simulink library "CartesianLib"  (R2024a)
settings: Solver=VariableStepAuto  StartTime=0.0  StopTime=10.0  RelTol=1e-3
undefined symbols (not defined in the file): X, Y, Z
libraries: sm_lib x43
(part 1 of 2)
settings Model: Creator=abirdas  LastModifiedBy=abirdas

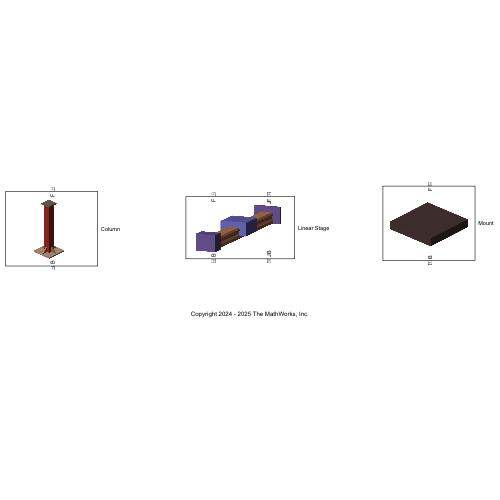
[thumbnail: Simulink's stored preview of the top-level diagram]
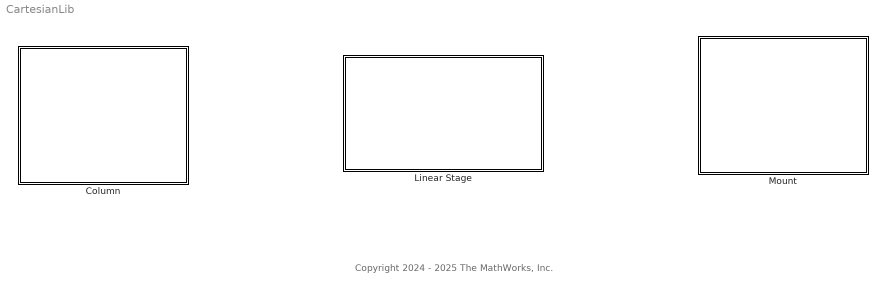
== system CartesianLib ==
  note: Copyright 2024 - 2025 The MathWorks, Inc.
  Column : Subsystem  mask(Column){lengthColumn=0.2, widthColumn=0.02, typeInertiaColumn=Calculate from Geometry, densityColumn=7780, massColumn=1, CMColumn=[0 0 0], MOIColumn=[1 1 1], POIColumn=[0 0 0], colorColumn=[0.8 0.2 0.2]}
      mask prompts: lengthColumn "Column length (m)"; widthColumn "Column width (m)"; typeInertiaColumn "Inertia type"; densityColumn "Density (kg/m^3)"; massColumn "Mass (kg)"; CMColumn "Center of mass (m)"; MOIColumn "Moments of inertia (kg/m^2)"; POIColumn "Products of inertia (kg/m^2)"; colorColumn "Column color"
      mask help:
      | Consists of a bottom plate, a pillar, a top plate and four gusset plates. These components are rigidly connected to one another.
      |
      | Attachment points are:
      | B: Body frame located at the centroid of the bottom surface of the bottom plate of the column.
      | F: Body frame located at the centroid of the top surface of the top plate of the column.
      |
      | Where
      | Column length: Length of the vertical pillar
      | Column width: Width of the vertical pillar
      mask init:
      | % Vertices of gusset plate
      | v1 = [0, 0];
      | v2 = [0.8*widthColumn, 0];
      | v3 = [0, 0.8*widthColumn];
      | sectionGusset = [v1; v2; v3];
      settings: PortSchema="{\"entries\":[{\"content\":{\"sides\":[{\"content\":{},\"type\":\"ConnectorPlacement.EquallySpacedRectSide\",\"uuid\":\"5b485af5-4f05-4248-a7f3-08377bf9cff2\"},{\"content\":{\"side\":\"RIGHT\"},\"type\":\"ConnectorPlacement.EquallySpacedRectSide\",\"uuid\":\"824380b3-967b-4422-aed9-09760effc9b4\"},{\"content\":{\"connectorIds\":[\"LConn1\"],\"side\":\"TOP\"},\"type\":\"ConnectorPlacement.EquallySpacedRectSide\",\"uuid\":\"4c7d634e-a270-49ee-a9b6-ce866eb97663\"},{\"content\":{\"connectorIds\":[\"RConn1\"],\"side\":\"BOTTOM\"},\"type\":\"ConnectorPlacement.EquallySpacedRectSide\",\"uuid\":\"85de5209-dd21-416e-83dd-d7e9fdf0c122\"}]},\"type\":\"ConnectorPlacement.EquallySpacedConnector\",\"uuid\":\"704e5fa1-0bef-4b5b-a1a4-570354550c26\"}],\"packageUris\":[\"http://schema.mathworks.com/mf0/Connector/R2020b\"],\"version\":\"1.0\"}"
      mask Help: web('DocumentationColumn.html')
      mask Callback typeInertiaColumn:
      | maskObj = Simulink.Mask.get(gcb);
      | typeInertiaColumn = maskObj.getParameter('typeInertiaColumn');
      | massColumn = maskObj.getParameter('massColumn');
      | CMColumn = maskObj.getParameter('CMColumn');
      | MOIColumn = maskObj.getParameter('MOIColumn');
      | POIColumn = maskObj.getParameter('POIColumn');
      | densityColumn = maskObj.getParameter('densityColumn');
      | basePlatePath = [gcb,'/Base Plate'];
      | pillarPath = [gcb,'/Pillar'];
      | topPlatePath = [gcb,'/Top Plate'];
      | gusset1Path = [gcb,'/Gusset plate1'];
      | gusset2Path = [gcb,'/Gusset plate2'];
      | gusset3Path = [gcb,'/Gusset plate3'];
      | gusset4Path = [gcb,'/Gusset plate4'];
      | 
      | if strcmp(typeInertiaColumn.Value,'Calculate from Geometry')
      |     massColumn.Visible='off';
      |     CMColumn.Visible='off';
      |     MOIColumn.Visible='off';
      |     POIColumn.Visible='off';
      |     densityColumn.Visible='on';
      |     set_param(basePlatePath,'InertiaType','CalculateFromGeometry');
      |     set_param(basePlatePath,'BasedOnType','Density');
      |     set_param(pillarPath,'InertiaType','CalculateFromGeometry');
      |     set_param(pillarPath,'BasedOnType','Density');
      |     set_param(topPlatePath,'InertiaType','CalculateFromGeometry');
      |     set_param(topPlatePath,'BasedOnType','Density');
      |     set_param(gusset1Path,'InertiaType','CalculateFromGeometry');
      |     set_param(gusset1Path,'BasedOnType','Density');
      |     set_param(gusset2Path,'InertiaType','CalculateFromGeometry');
      |     set_param(gusset2Path,'BasedOnType','Density');
      |     set_param(gusset3Path,'InertiaType','CalculateFromGeometry');
      |     set_param(gusset3Path,'BasedOnType','Density');
      |     set_param(gusset4Path,'InertiaType','CalculateFromGeometry');
      |     set_param(gusset4Path,'BasedOnType','Density');
      | elseif strcmp(typeInertiaColumn.Value,'Custom')
      |     massColumn.Visible='on';
      |     CMColumn.Visible='on';
      |     MOIColumn.Visible='on';
      |     POIColumn.Visible='on';
      |     densityColumn.Visible='off';
      |     set_param(basePlatePath,'InertiaType','Custom');
      |     set_param(pillarPath,'InertiaType','Custom');
      |     set_param(topPlatePath,'InertiaType','Custom');
      |     set_param(gusset1Path,'InertiaType','Custom');
      |     set_param(gusset2Path,'InertiaType','Custom');
      |     set_param(gusset3Path,'InertiaType','Custom');
      |     set_param(gusset4Path,'InertiaType','Custom');
      | end
      mask DialogControl Container1 Prompt: Geometry
      mask DialogControl Container2 Prompt: Inertia
      mask DialogControl Container3 Prompt: Graphic
      mask Display:
      | image('ColumnIcon.png');
      | port_label('rconn',1,'B');
      | port_label('lconn',1,'F');
  Linear Stage : Subsystem  mask(Linear Stage){systemGuide=Rail-block, axisGuide=X-axis, stroke=0.8, widthRail=0.05, diaScrew=0.05, typeInertiaGuide=Calculate from Geometry, densityGuide=7780, massGuide=1, CMGuide=[0 0 0], MOIGuide=[1 1 1], POIGuide=[0 0 0], typeInertiaCarriage=Calculate from Geometry, densityCarriage=7780, massCarriage=0.5, CMCarriage=[0 0 0], MOICarriage=[1 1 1], POICarriage=[0 0 0], colorGuide=[0.7 0.6 0.4], colorCarriage=[0.5 0.5 0.9]}
      mask prompts: systemGuide "Guide system"; axisGuide "Guide axis"; stroke "Maximum stroke (m)"; widthRail "Rail width (in m)"; diaScrew "Screw diameter (in m)"; typeInertiaGuide "Inertia type"; densityGuide "Density (kg/m^3)"; massGuide "Mass (kg)"; CMGuide "Center of mass (m)"; MOIGuide "Moments of inertia (kg*m^2)"; POIGuide "Products of inertia (kg*m^2)"; typeInertiaCarriage "Inertia type"; densityCarriage "Density (kg/m^3)"; massCarriage "Mass (kg)"; CMCarriage "Center of mass (m)"; MOICarriage "Moments of inertia (kg*m^2)"; POICarriage "Products of inertia (kg*m^2)"; colorGuide "Linear guide color"; colorCarriage "Carriage color"
      mask help:
      | Consists of a linear guide (fixed) and a carriage (moving). The carriage must be connected to the linear guide using a Prismatic Joint. The linear guide consists of a guide, a motor housing and a tail end plate. These components are rigidly connected to one another.
      |
      | Attachment points are:
      | B: Body frame located at the centroid of the bottom surface of the fixed linear guide.
      | F: Body frame located at the centroid of the top surface of the moving carriage.
      | JB: Body frame located at the centroid of the mating surface of the fixed linear guide (top surface of a rail or curved surface of a cylindrical lead screw).
      | JF: Body frame located at the centroid of the mating surface of the moving carriage (inner flat surface of a block or annular surface of a bearing).
      |
      | Guide system can be of following types:
      | Rail-block
      | Lead screw-bearing
      |
      | Where
      | Maximum stroke: Maximum stroke length of the moving carriage of the linear stage
      | Rail width: Width of the rail
      | Screw diameter: Diameter of the leadscrew
      mask init:
      | maskObj = Simulink.Mask.get(gcb);
      | strokeValue = get_param(gcb,'value@stroke');
      | diaScrewValue = get_param(gcb,'value@diaScrew');
      | widthRailValue = get_param(gcb,'value@widthRail');
      | guideSystemPath = [gcb,'/Linear Guide'];
      | carriageSystemPath = [gcb,'/Carriage'];
      | fracLengthCarriageGuide = 0.2;
      | lengthRail = strokeValue/(1-fracLengthCarriageGuide);
      | lengthBlock = fracLengthCarriageGuide*lengthRail;
      | lengthScrew = strokeValue/(1-fracLengthCarriageGuide);
      | lengthBearing = fracLengthCarriageGuide*lengthScrew;
      | widthBearing = 2*diaScrewValue;
      | set_param(guideSystemPath,'lengthRail',num2str(lengthRail));
      | set_param(carriageSystemPath,'lengthBlock',num2str(lengthBlock));
      | set_param(guideSystemPath,'lengthScrew',num2str(lengthScrew));
      | set_param(carriageSystemPath,'lengthBearing',num2str(lengthBearing));
      | set_param(carriageSystemPath,'widthBearing',num2str(widthBearing));
      settings: PortSchema="{\"entries\":[{\"content\":{\"sides\":[{\"content\":{},\"type\":\"ConnectorPlacement.EquallySpacedRectSide\",\"uuid\":\"d53cf38a-f5b3-47f8-82db-beff20fa4a2b\"},{\"content\":{\"side\":\"RIGHT\"},\"type\":\"ConnectorPlacement.EquallySpacedRectSide\",\"uuid\":\"94dfc98b-3b78-4115-aa23-28a77ecd38e0\"},{\"content\":{\"connectorIds\":[\"LConn1\",\"LConn2\"],\"side\":\"TOP\"},\"type\":\"ConnectorPlacement.EquallySpacedRectSide\",\"uuid\":\"e4fbd77d-7bbf-4148-915b-f65068a9f00f\"},{\"content\":{\"connectorIds\":[\"RConn1\",\"RConn2\"],\"side\":\"BOTTOM\"},\"type\":\"ConnectorPlacement.EquallySpacedRectSide\",\"uuid\":\"2c4cbc2f-3e02-45ca-a613-d08563667735\"}]},\"type\":\"ConnectorPlacement.EquallySpacedConnector\",\"uuid\":\"e420e2db-418c-4d14-b432-78e557ce3d1e\"}],\"packageUris\":[\"http://schema.mathworks.com/mf0/Connector/R2020b\"],\"version\":\"1.0\"}"
      mask Help: web('DocumentationLinearStage.html')
      mask TypeOptions systemGuide: Rail-block | Lead screw-bearing
      mask Callback systemGuide: LinearStageMask
      mask Callback axisGuide: LinearStageMask
      mask TypeOptions widthRail: Linear Guide/widthRail
      mask TypeOptions diaScrew: Linear Guide/diaShaft
      mask Callback typeInertiaGuide: LinearStageMask
      mask Callback typeInertiaCarriage: LinearStageMask
      mask DialogControl Container1 Prompt: Configuration
      mask DialogControl Container2 Prompt: Geometry
      mask DialogControl Container3 Prompt: Inertia
      mask DialogControl Guide Prompt: Linear Guide
      mask DialogControl Carriage Prompt: Carriage
      mask DialogControl Container4 Prompt: Graphic
      mask Display:
      | image('LinearStageIcon.png');
      | port_label('rconn',1,'B');
      | port_label('lconn',1,'F');
      | port_label('rconn',2,'JB');
      | port_label('lconn',2,'JF');
  Mount : Subsystem  mask(Mount){typeMount=Plate mount, widthMount=0.05, angleMount=45, angleRotate=0, typeInertiaMount=Calculate from Geometry, densityMount=7780, massMount=0.1, CMMount=[0 0 0], MOIMount=[1 1 1], POIMount=[0 0 0], colorMount=[0.35 0.25 0.25]}
      mask prompts: typeMount "Mount type"; widthMount "Mount width (m)"; angleMount "Mount angle (deg)"; angleRotate "Rotation angle about mount base (deg)"; typeInertiaMount "Inertia type"; densityMount "Density (kg/m^3)"; massMount "Mass (kg)"; CMMount "Center of mass (m)"; MOIMount "Moments of inertia (kg/m^2)"; POIMount "Products of inertia (kg/m^2)"; colorMount "Mount color"
      mask help:
      | Mount block models the rigid body structural component in a Cartesian robot that supports a linear stage.
      |
      | Attachment points are:
      | B: Body frame located at the centroid of the bottom surface of the mount.
      | F: Body frame located at the centroid of the top or side surface of the mount.
      |
      | Mount can be of following types:
      | Plate mount
      | L-shaped mount
      | Angle mount
      |
      | Where
      | Mount width: Width of the mount.
      | Mount angle: Angle of the side surface of the mount relative to the bottom surface.
      | Rotation angle about mount base: Angle of rotation of the mount about perpendicular to the bottom surface.
      mask init:
      | maskObj = Simulink.Mask.get(gcb);
      | typeMountObj = maskObj.getParameter('typeMount');
      | widthMountObj = maskObj.getParameter('widthMount');
      | angleMountObj = maskObj.getParameter('angleMount');
      | angleRotateObj = maskObj.getParameter('angleRotate');
      | 
      | wMount = get_param(gcb,'value@widthMount');
      | tMount = wMount/20; % Mount thickness assumed
      | angleMountValue = get_param(gcb,'value@angleMount');
      | 
      | mountSystemPath = [gcb,'/Mount System'];
      | set_param(mountSystemPath,'typeMount',typeMountObj.Value);
      | set_param(mountSystemPath,'widthMount',widthMountObj.Value);
      | set_param(mountSystemPath,'angleMount',angleMountObj.Value);
      | set_param(mountSystemPath,'angleRotate',angleRotateObj.Value);
      | 
      | % Vertices and sectional area for L-shaped mount
      | vL1 = [wMount, tMount];
      | vL2 = [wMount, 0];
      | vL3 = [0, 0];
      | vL4 = [0, wMount];
      | vL5 = [tMount, wMount];
      | vL6 = [tMount, tMount];
      | sectionLMount = flipud([vL1; vL2; vL3; vL4; vL5; vL6]);
      | 
      | % Vertices and sectional area for angle mount
      | theta = pi/180*angleMountValue;
      | vA1 = [wMount, tMount];
      | vA2 = [wMount, 0];
      | vA3 = [0, 0];
      | vA4 = [wMount*cos(theta), wMount*sin(theta)];
      | vA5 = [wMount*cos(theta) + tMount*sin(theta), ...
      |     wMount*sin(theta) - tMount*cos(theta)];
      | vA6 = [tMount/sin(0.5*theta), tMount];
      | sectionAngleMount = flipud([vA1; vA2; vA3; vA4; vA5; vA6]);
      settings: PortSchema="{\"entries\":[{\"content\":{\"sides\":[{\"content\":{},\"type\":\"ConnectorPlacement.EquallySpacedRectSide\",\"uuid\":\"5b485af5-4f05-4248-a7f3-08377bf9cff2\"},{\"content\":{\"side\":\"RIGHT\"},\"type\":\"ConnectorPlacement.EquallySpacedRectSide\",\"uuid\":\"824380b3-967b-4422-aed9-09760effc9b4\"},{\"content\":{\"connectorIds\":[\"LConn1\"],\"side\":\"TOP\"},\"type\":\"ConnectorPlacement.EquallySpacedRectSide\",\"uuid\":\"4c7d634e-a270-49ee-a9b6-ce866eb97663\"},{\"content\":{\"connectorIds\":[\"RConn1\"],\"side\":\"BOTTOM\"},\"type\":\"ConnectorPlacement.EquallySpacedRectSide\",\"uuid\":\"cf1b7e56-31ef-45be-a1b8-627d18404b66\"}]},\"type\":\"ConnectorPlacement.EquallySpacedConnector\",\"uuid\":\"704e5fa1-0bef-4b5b-a1a4-570354550c26\"}],\"packageUris\":[\"http://schema.mathworks.com/mf0/Connector/R2020b\"],\"version\":\"1.0\"}"
      mask Help: web('DocumentationMount.html')
      mask Callback typeMount:
      | maskObj = Simulink.Mask.get(gcb);
      | typeMount = maskObj.getParameter('typeMount');
      | widthMount = maskObj.getParameter('widthMount');
      | angleMount = maskObj.getParameter('angleMount');
      | angleRotate = maskObj.getParameter('angleRotate');
      | mountSystemPath = [gcb,'/Mount System'];
      | transform1Path = [gcb,'/Rigid Transform1'];
      | transform2Path = [gcb,'/Rigid Transform4'];
      | angleRotateValue = angleRotate.Value;
      | 
      | if strcmp(typeMount.Value,'Plate mount')
      |     widthMount.Visible = 'on';
      |     angleMount.Visible = 'off';
      |     angleRotate.Visible = 'off';
      |     set_param(mountSystemPath, 'LabelModeActiveChoice', 'PlateMount');
      |     set_param(transform1Path, 'RotationSequenceAngles', '[0 0 0]');
      |     set_param(transform2Path, 'RotationSequenceAngles', '[0 0 0]');
      | elseif strcmp(typeMount.Value,'L-shaped mount')
      |     widthMount.Visible = 'on';
      |     angleMount.Visible = 'off';
      |     angleRotate.Visible = 'on';
      |     set_param(mountSystemPath, 'LabelModeActiveChoice', 'LMount');
      |     set_param(transform1Path, 'RotationSequenceAngles', '[90 0 180]');
      |     set_param(transform2Path, 'RotationSequenceAngles', '[90 0 180]');
      | elseif strcmp(typeMount.Value,'Angle mount')
      |     widthMount.Visible = 'on';
      |     angleMount.Visible = 'on';
      |     angleRotate.Visible = 'on';
      |     set_param(mountSystemPath, 'LabelModeActiveChoice', 'AngleMount');
      |     set_param(transform1Path, 'RotationSequenceAngles', '[90 0 180]');
      |     set_param(transform2Path, 'RotationSequenceAngles', '[90 0 180]');
      | end
      mask Callback typeInertiaMount:
      | maskObj = Simulink.Mask.get(gcb);
      | typeInertiaMount = maskObj.getParameter('typeInertiaMount');
      | massMount = maskObj.getParameter('massMount');
      | CMMount = maskObj.getParameter('CMMount');
      | MOIMount = maskObj.getParameter('MOIMount');
      | POIMount = maskObj.getParameter('POIMount');
      | densityMount = maskObj.getParameter('densityMount');
      | plateMountPath = [gcb,'/Mount System/Plate Mount/Brick Solid'];
      | LMountPath = [gcb,'/Mount System/L-Shaped Mount/Extruded Solid'];
      | angleMountPath = [gcb,'/Mount System/Angle Mount/Extruded Solid'];
      | 
      | if strcmp(typeInertiaMount.Value,'Calculate from Geometry')
      |     massMount.Visible='off';
      |     CMMount.Visible='off';
      |     MOIMount.Visible='off';
      |     POIMount.Visible='off';
      |     densityMount.Visible='on';
      |     set_param(plateMountPath,'InertiaType','CalculateFromGeometry');
      |     set_param(plateMountPath,'BasedOnType','Density');
      |     set_param(LMountPath,'InertiaType','CalculateFromGeometry');
      |     set_param(LMountPath,'BasedOnType','Density');
      |     set_param(angleMountPath,'InertiaType','CalculateFromGeometry');
      |     set_param(angleMountPath,'BasedOnType','Density');
      | elseif strcmp(typeInertiaMount.Value,'Custom')
      |     massMount.Visible='on';
      |     CMMount.Visible='on';
      |     MOIMount.Visible='on';
      |     POIMount.Visible='on';
      |     densityMount.Visible='off';
      |     set_param(plateMountPath,'InertiaType','Custom');
      |     set_param(LMountPath,'InertiaType','Custom');
      |     set_param(angleMountPath,'InertiaType','Custom');
      | end
      mask DialogControl Container1 Prompt: Configuration
      mask DialogControl Container2 Prompt: Geometry
      mask DialogControl Container3 Prompt: Inertia
      mask DialogControl Container6 Prompt: Graphic
      mask Display:
      | image('PlateMountIcon.png');
      | port_label('rconn',1,'B');
      | port_label('lconn',1,'F');

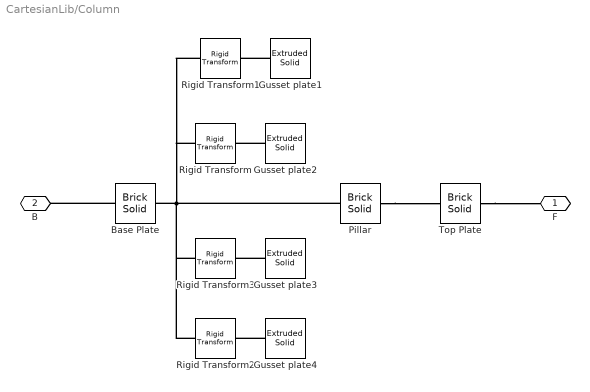
== system CartesianLib/Column ==
  Base Plate : sm_lib/Body Elements/Brick Solid  BrickDimensions=[3*widthColumn 3*widthColumn 0.2*widthColumn]  BrickDimensionsUnits=m  ExportEntireGeometry=off  InertiaType=CalculateFromGeometry  BasedOnType=Density  Density=densityColumn  DensityUnits=kg/m^3  Mass=0  MassUnits=kg  CenterOfMass=[0 0 0]  CenterOfMassUnits=m  MomentsOfInertia=[0 0 0]  MomentsOfInertiaUnits=kg*m^2  ProductsOfInertia=[0 0 0]  ProductsOfInertiaUnits=kg*m^2  GraphicType=FromGeometry  MarkerShape=Sphere  MarkerSize=10  GraphicVisPropType=SimpleVisualProperties  GraphicDiffuseColor=[0.9 0.7 0.6]  GraphicOpacity=1  GraphicSpecularColor=[0.5 0.5 0.5 1.0]  GraphicAmbientColor=[0.15 0.15 0.15 1.0]  GraphicEmissiveColor=[0.0 0.0 0.0 1.0]  GraphicShininess=75  DoExposeReferenceFrame=off  SerializedFrames=<Frames><Frame><Id>Frame1</Id><Value><Name>F1</Name><Origin><Source>GeometricFeature</Source><FeatureName>-z surface</FeatureName></Origin><PrimaryAxis><DefinedDirection>+Z</DefinedDirection><Source>ReferenceFrame</Source><SourceDirection>+Z</SourceDirection><FeatureName></FeatureName></PrimaryAxis><SecondaryAxis><DefinedDirection>+X</DefinedDirection><Source>ReferenceFrame</Source><SourceDirection>+X</SourceDirection><FeatureName></FeatureName></SecondaryAxis></Value></Frame><Frame><Id>Frame2</Id><Value><Name>F2</Name><Origin><Source>GeometricFeature</Source><FeatureName>+z surface</FeatureName></Origin><PrimaryAxis><DefinedDirection>+Z</DefinedDirection><Source>ReferenceFrame</Source><SourceDirection>+Z</SourceDirection><FeatureName></FeatureName></PrimaryAxis><SecondaryAxis><DefinedDirection>+X</DefinedDirection><Source>ReferenceFrame</Source><SourceDirection>+X</SourceDirection><FeatureName></FeatureName></SecondaryAxis></Value></Frame></Frames>
  Gusset plate{1..4} (4 alike) : sm_lib/Body Elements/Extruded Solid  ExtrusionType=General  PolygonNumSides=3  PolygonOuterRadius=0.8*widthColumn  PolygonOuterRadiusUnits=m  ExportEntireGeometry=off  ExtrusionCrossSection=sectionGusset  ExtrusionCrossSectionUnits=m  ExportConvexHullGeometry=off  ExtrusionLength=0.2*widthColumn  ExtrusionLengthUnits=m  InertiaType=CalculateFromGeometry  BasedOnType=Density  Density=densityColumn  DensityUnits=kg/m^3  Mass=0  MassUnits=kg  CenterOfMass=[0 0 0]  CenterOfMassUnits=m  MomentsOfInertia=[0 0 0]  MomentsOfInertiaUnits=kg*m^2  ProductsOfInertia=[0 0 0]  ProductsOfInertiaUnits=kg*m^2  GraphicType=FromGeometry  MarkerShape=Sphere  MarkerSize=10  GraphicVisPropType=SimpleVisualProperties  GraphicDiffuseColor=[0.7 0.6 0.4]  GraphicOpacity=1  GraphicSpecularColor=[0.5 0.5 0.5 1.0]  GraphicAmbientColor=[0.15 0.15 0.15 1.0]  GraphicEmissiveColor=[0.0 0.0 0.0 1.0]  GraphicShininess=75  DoExposeReferenceFrame=off  SerializedFrames=<Frames><Frame><Id>Frame1</Id><Value><Name>F1</Name><Origin><Source>GeometricFeature</Source><FeatureName>side surface 1</FeatureName></Origin><PrimaryAxis><DefinedDirection>+Z</DefinedDirection><Source>ReferenceFrame</Source><SourceDirection>+Z</SourceDirection><FeatureName></FeatureName></PrimaryAxis><SecondaryAxis><DefinedDirection>+X</DefinedDirection><Source>ReferenceFrame</Source><SourceDirection>+X</SourceDirection><FeatureName></FeatureName></SecondaryAxis></Value></Frame></Frames>
  Pillar : sm_lib/Body Elements/Brick Solid  BrickDimensions="[widthColumn widthColumn  lengthColumn]"  BrickDimensionsUnits=m  ExportEntireGeometry=off  InertiaType=CalculateFromGeometry  BasedOnType=Density  Density=densityColumn  DensityUnits=kg/m^3  Mass=massColumn  MassUnits=kg  CenterOfMass=CMColumn  CenterOfMassUnits=m  MomentsOfInertia=MOIColumn  MomentsOfInertiaUnits=kg*m^2  ProductsOfInertia=POIColumn  ProductsOfInertiaUnits=kg*m^2  GraphicType=FromGeometry  MarkerShape=Sphere  MarkerSize=10  GraphicVisPropType=SimpleVisualProperties  GraphicDiffuseColor=colorColumn  GraphicOpacity=1  GraphicSpecularColor=[0.5 0.5 0.5 1.0]  GraphicAmbientColor=[0.15 0.15 0.15 1.0]  GraphicEmissiveColor=[0.0 0.0 0.0 1.0]  GraphicShininess=75  DoExposeReferenceFrame=off  SerializedFrames=<Frames><Frame><Id>Frame1</Id><Value><Name>F1</Name><Origin><Source>GeometricFeature</Source><FeatureName>-z surface</FeatureName></Origin><PrimaryAxis><DefinedDirection>+Z</DefinedDirection><Source>ReferenceFrame</Source><SourceDirection>+Z</SourceDirection><FeatureName></FeatureName></PrimaryAxis><SecondaryAxis><DefinedDirection>+X</DefinedDirection><Source>ReferenceFrame</Source><SourceDirection>+X</SourceDirection><FeatureName></FeatureName></SecondaryAxis></Value></Frame><Frame><Id>Frame2</Id><Value><Name>F2</Name><Origin><Source>GeometricFeature</Source><FeatureName>+z surface</FeatureName></Origin><PrimaryAxis><DefinedDirection>+Z</DefinedDirection><Source>ReferenceFrame</Source><SourceDirection>+Z</SourceDirection><FeatureName></FeatureName></PrimaryAxis><SecondaryAxis><DefinedDirection>+X</DefinedDirection><Source>ReferenceFrame</Source><SourceDirection>+X</SourceDirection><FeatureName></FeatureName></SecondaryAxis></Value></Frame></Frames>
  Rigid Transform : sm_lib/Frames and Transforms/Rigid Transform  RotationMethod=StandardAxis  FollAlignAxisA=+X  BaseAlignAxisA=+Y  FollAlignAxisB=+Y  BaseAlignAxisB=+Z  RotationStandardAxis=+X  RotationAngle=90  RotationAngleUnits=deg  RotationArbitraryAxis=[0 0 1]  RotationSequenceAxes=FollowerAxes  RotationSequence=XYX  RotationSequenceAngles=[0 0 0]  RotationSequenceAnglesUnits=deg  RotationMatrix=[1 0 0;0 1 0;0 0 1]  Quaternion=[1 0 0 0]  TranslationMethod=StandardAxis  TranslationCartesianOffset=[0 0 0]  TranslationCartesianOffsetUnits=m  TranslationStandardAxis=+X  TranslationStandardOffset=0.9*widthColumn  TranslationStandardOffsetUnits=m  TranslationROffset=0  TranslationROffsetUnits=m  TranslationThetaOffset=0  TranslationThetaOffsetUnits=deg  TranslationZOffset=0  TranslationZOffsetUnits=m
  Rigid Transform1 : sm_lib/Frames and Transforms/Rigid Transform  RotationMethod=RotationSequence  FollAlignAxisA=+X  BaseAlignAxisA=+Y  FollAlignAxisB=+Y  BaseAlignAxisB=+Z  RotationStandardAxis=+X  RotationAngle=90  RotationAngleUnits=deg  RotationArbitraryAxis=[0 0 1]  RotationSequenceAxes=BaseAxes  RotationSequence=XYZ  RotationSequenceAngles=[90 0 90]  RotationSequenceAnglesUnits=deg  RotationMatrix=[1 0 0;0 1 0;0 0 1]  Quaternion=[1 0 0 0]  TranslationMethod=StandardAxis  TranslationCartesianOffset=[0 0 0]  TranslationCartesianOffsetUnits=m  TranslationStandardAxis=+Y  TranslationStandardOffset=0.9*widthColumn  TranslationStandardOffsetUnits=m  TranslationROffset=0  TranslationROffsetUnits=m  TranslationThetaOffset=0  TranslationThetaOffsetUnits=deg  TranslationZOffset=0  TranslationZOffsetUnits=m
  Rigid Transform2 : sm_lib/Frames and Transforms/Rigid Transform  RotationMethod=RotationSequence  FollAlignAxisA=+X  BaseAlignAxisA=+Y  FollAlignAxisB=+Y  BaseAlignAxisB=+Z  RotationStandardAxis=-X  RotationAngle=90  RotationAngleUnits=deg  RotationArbitraryAxis=[0 0 1]  RotationSequenceAxes=BaseAxes  RotationSequence=XYZ  RotationSequenceAngles=[90 0 180]  RotationSequenceAnglesUnits=deg  RotationMatrix=[1 0 0;0 1 0;0 0 1]  Quaternion=[1 0 0 0]  TranslationMethod=StandardAxis  TranslationCartesianOffset=[0 0 0]  TranslationCartesianOffsetUnits=m  TranslationStandardAxis=-X  TranslationStandardOffset=0.9*widthColumn  TranslationStandardOffsetUnits=m  TranslationROffset=0  TranslationROffsetUnits=m  TranslationThetaOffset=0  TranslationThetaOffsetUnits=deg  TranslationZOffset=0  TranslationZOffsetUnits=m
  Rigid Transform3 : sm_lib/Frames and Transforms/Rigid Transform  RotationMethod=RotationSequence  FollAlignAxisA=+X  BaseAlignAxisA=+Y  FollAlignAxisB=+Y  BaseAlignAxisB=+Z  RotationStandardAxis=+X  RotationAngle=90  RotationAngleUnits=deg  RotationArbitraryAxis=[0 0 1]  RotationSequenceAxes=BaseAxes  RotationSequence=XYZ  RotationSequenceAngles=[90 0 -90]  RotationSequenceAnglesUnits=deg  RotationMatrix=[1 0 0;0 1 0;0 0 1]  Quaternion=[1 0 0 0]  TranslationMethod=StandardAxis  TranslationCartesianOffset=[0 0 0]  TranslationCartesianOffsetUnits=m  TranslationStandardAxis=-Y  TranslationStandardOffset=0.9*widthColumn  TranslationStandardOffsetUnits=m  TranslationROffset=0  TranslationROffsetUnits=m  TranslationThetaOffset=0  TranslationThetaOffsetUnits=deg  TranslationZOffset=0  TranslationZOffsetUnits=m
  Top Plate : sm_lib/Body Elements/Brick Solid  BrickDimensions=[1.5*widthColumn 1.5*widthColumn 0.2*widthColumn]  BrickDimensionsUnits=m  ExportEntireGeometry=off  InertiaType=CalculateFromGeometry  BasedOnType=Density  Density=densityColumn  DensityUnits=kg/m^3  Mass=0  MassUnits=kg  CenterOfMass=[0 0 0]  CenterOfMassUnits=m  MomentsOfInertia=[0 0 0]  MomentsOfInertiaUnits=kg*m^2  ProductsOfInertia=[0 0 0]  ProductsOfInertiaUnits=kg*m^2  GraphicType=FromGeometry  MarkerShape=Sphere  MarkerSize=10  GraphicVisPropType=SimpleVisualProperties  GraphicDiffuseColor=[0.55 0.45 0.45]  GraphicOpacity=1  GraphicSpecularColor=[0.5 0.5 0.5 1.0]  GraphicAmbientColor=[0.15 0.15 0.15 1.0]  GraphicEmissiveColor=[0.0 0.0 0.0 1.0]  GraphicShininess=75  DoExposeReferenceFrame=off  SerializedFrames=<Frames><Frame><Id>Frame1</Id><Value><Name>F1</Name><Origin><Source>GeometricFeature</Source><FeatureName>-z surface</FeatureName></Origin><PrimaryAxis><DefinedDirection>+Z</DefinedDirection><Source>ReferenceFrame</Source><SourceDirection>+Z</SourceDirection><FeatureName></FeatureName></PrimaryAxis><SecondaryAxis><DefinedDirection>+X</DefinedDirection><Source>ReferenceFrame</Source><SourceDirection>+X</SourceDirection><FeatureName></FeatureName></SecondaryAxis></Value></Frame><Frame><Id>Frame2</Id><Value><Name>F2</Name><Origin><Source>GeometricFeature</Source><FeatureName>+z surface</FeatureName></Origin><PrimaryAxis><DefinedDirection>+Z</DefinedDirection><Source>ReferenceFrame</Source><SourceDirection>+Z</SourceDirection><FeatureName></FeatureName></PrimaryAxis><SecondaryAxis><DefinedDirection>+X</DefinedDirection><Source>ReferenceFrame</Source><SourceDirection>+X</SourceDirection><FeatureName></FeatureName></SecondaryAxis></Value></Frame></Frames>
  F : PMIOPort  Side=Left
  B : PMIOPort  Port=2  Side=Right
  connections:
  Base Plate/LConn1 -- B/RConn1
  Pillar/RConn1 -- Top Plate/LConn1
  Pillar/LConn1 -- Rigid Transform3/LConn1 -- Rigid Transform2/LConn1 -- Rigid Transform1/LConn1 -- Rigid Transform/LConn1 -- Base Plate/RConn1
  Top Plate/RConn1 -- F/RConn1
  Gusset plate2/LConn1 -- Rigid Transform/RConn1
  Gusset plate1/LConn1 -- Rigid Transform1/RConn1
  Gusset plate4/LConn1 -- Rigid Transform2/RConn1
  Gusset plate3/LConn1 -- Rigid Transform3/RConn1

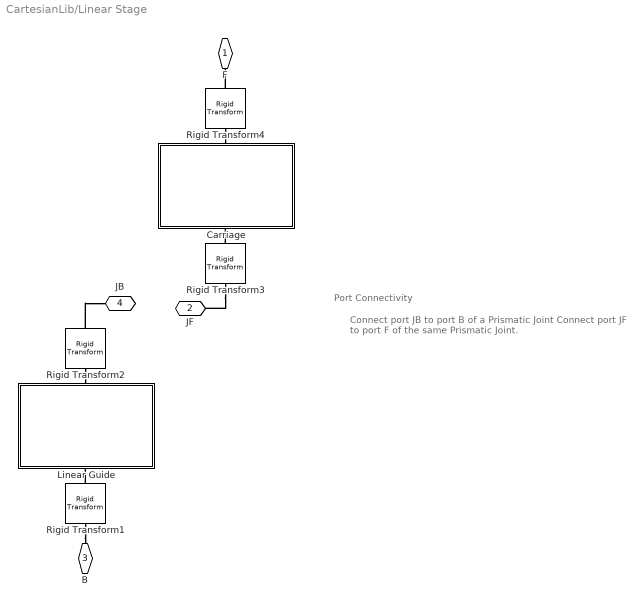
== system CartesianLib/Linear Stage ==
  note: Port Connectivity
  note: Connect port JB to port B of a Prismatic Joint
      | Connect port JF to port F of the same Prismatic Joint.
  Carriage : Subsystem  Variant=on  VariantControlMode=label  LabelModeActiveChoice=Block  mask{typeCarriage=Block, lengthBlock=0.2, widthSlideSurface=widthRail, lengthBearing=0.2, widthBearing=0.1}
      mask prompts: typeCarriage "Carriage type"; lengthBlock "Block length (m)"; widthSlideSurface "Sliding surface width (m)"; lengthBearing "Bearing length (m)"; widthBearing "Bearing width (m)"
      settings: PortSchema="{\"entries\":[{\"content\":{\"sides\":[{\"content\":{},\"type\":\"ConnectorPlacement.EquallySpacedRectSide\",\"uuid\":\"5b485af5-4f05-4248-a7f3-08377bf9cff2\"},{\"content\":{\"side\":\"RIGHT\"},\"type\":\"ConnectorPlacement.EquallySpacedRectSide\",\"uuid\":\"824380b3-967b-4422-aed9-09760effc9b4\"},{\"content\":{\"connectorIds\":[\"LConn1\"],\"side\":\"TOP\"},\"type\":\"ConnectorPlacement.EquallySpacedRectSide\",\"uuid\":\"4c7d634e-a270-49ee-a9b6-ce866eb97663\"},{\"content\":{\"connectorIds\":[\"RConn1\"],\"side\":\"BOTTOM\"},\"type\":\"ConnectorPlacement.EquallySpacedRectSide\",\"uuid\":\"cfbd31b8-7d97-48d4-9fa2-7fcdf344ca09\"}]},\"type\":\"ConnectorPlacement.EquallySpacedConnector\",\"uuid\":\"704e5fa1-0bef-4b5b-a1a4-570354550c26\"}],\"packageUris\":[\"http://schema.mathworks.com/mf0/Connector/R2020b\"],\"version\":\"1.0\"}"
      mask TypeOptions typeCarriage: Block | Bearing
      mask Callback typeCarriage:
      | maskObj = Simulink.Mask.get(gcb);
      | typeCarriage = maskObj.getParameter('typeCarriage');
      | lengthBlock = maskObj.getParameter('lengthBlock');
      | widthSlideSurface = maskObj.getParameter('widthSlideSurface');
      | lengthBearing = maskObj.getParameter('lengthBearing');
      | widthBearing = maskObj.getParameter('widthBearing');
      | blockPath = gcb;
      | if strcmp(typeCarriage.Value,'Block')
      |     lengthBlock.Visible = 'on';
      |     widthSlideSurface.Visible = 'on';
      |     lengthBearing.Visible = 'off';
      |     widthBearing.Visible = 'off';
      |     set_param(blockPath, 'LabelModeActiveChoice', 'Block');
      | elseif strcmp(typeCarriage.Value,'Bearing')
      |     lengthBlock.Visible = 'off';
      |     widthSlideSurface.Visible = 'off';
      |     lengthBearing.Visible = 'on';
      |     widthBearing.Visible = 'on';
      |     set_param(blockPath, 'LabelModeActiveChoice', 'Bearing');
      | end
  Linear Guide : Subsystem  Variant=on  VariantControlMode=label  LabelModeActiveChoice=Rail  mask{typeGuide=Rail, lengthRail=1, widthRail=widthRail, lengthScrew=1, diaScrew=diaScrew}
      mask prompts: typeGuide "Guide type"; lengthRail "Rail length (m)"; widthRail "Rail width (m)"; lengthScrew "Screw length (m)"; diaScrew "Screw diameter (m)"
      settings: PortSchema="{\"entries\":[{\"content\":{\"sides\":[{\"content\":{},\"type\":\"ConnectorPlacement.EquallySpacedRectSide\",\"uuid\":\"5b485af5-4f05-4248-a7f3-08377bf9cff2\"},{\"content\":{\"side\":\"RIGHT\"},\"type\":\"ConnectorPlacement.EquallySpacedRectSide\",\"uuid\":\"824380b3-967b-4422-aed9-09760effc9b4\"},{\"content\":{\"connectorIds\":[\"LConn1\"],\"side\":\"TOP\"},\"type\":\"ConnectorPlacement.EquallySpacedRectSide\",\"uuid\":\"4c7d634e-a270-49ee-a9b6-ce866eb97663\"},{\"content\":{\"connectorIds\":[\"RConn1\"],\"side\":\"BOTTOM\"},\"type\":\"ConnectorPlacement.EquallySpacedRectSide\",\"uuid\":\"90343422-ff8b-4fea-97fe-73f039a54ffa\"}]},\"type\":\"ConnectorPlacement.EquallySpacedConnector\",\"uuid\":\"704e5fa1-0bef-4b5b-a1a4-570354550c26\"}],\"packageUris\":[\"http://schema.mathworks.com/mf0/Connector/R2020b\"],\"version\":\"1.0\"}"
      mask TypeOptions typeGuide: Rail | Lead screw
      mask Callback typeGuide:
      | maskObj = Simulink.Mask.get(gcb);
      | typeGuide = maskObj.getParameter('typeGuide');
      | lengthRail = maskObj.getParameter('lengthRail');
      | widthRail = maskObj.getParameter('widthRail');
      | lengthScrew = maskObj.getParameter('lengthScrew');
      | diaScrew = maskObj.getParameter('diaScrew');
      | blockPath = gcb;
      | if strcmp(typeGuide.Value,'Rail')
      |     lengthRail.Visible = 'on';
      |     widthRail.Visible = 'on';
      |     lengthScrew.Visible = 'off';
      |     diaScrew.Visible = 'off';
      |     set_param(blockPath, 'LabelModeActiveChoice', 'Rail');
      | elseif strcmp(typeGuide.Value,'Lead screw')
      |     lengthRail.Visible = 'off';
      |     widthRail.Visible = 'off';
      |     lengthScrew.Visible = 'on';
      |     diaScrew.Visible = 'on';
      |     set_param(blockPath, 'LabelModeActiveChoice', 'Screw');
      | end
  Rigid Transform1 : sm_lib/Frames and Transforms/Rigid Transform  RotationMethod=RotationSequence  FollAlignAxisA=+X  BaseAlignAxisA=+Y  FollAlignAxisB=+Y  BaseAlignAxisB=+Z  RotationStandardAxis=+Z  RotationAngle=-90  RotationAngleUnits=deg  RotationArbitraryAxis=[0 0 1]  RotationSequenceAxes=BaseAxes  RotationSequence=ZYX  RotationSequenceAngles=[90 90 0]  RotationSequenceAnglesUnits=deg  RotationMatrix=[1 0 0;0 1 0;0 0 1]  Quaternion=[1 0 0 0]  TranslationMethod=None  TranslationCartesianOffset=[0 0 0]  TranslationCartesianOffsetUnits=m  TranslationStandardAxis=+Z  TranslationStandardOffset=0  TranslationStandardOffsetUnits=m  TranslationROffset=0  TranslationROffsetUnits=m  TranslationThetaOffset=0  TranslationThetaOffsetUnits=deg  TranslationZOffset=0  TranslationZOffsetUnits=m
  Rigid Transform2 : sm_lib/Frames and Transforms/Rigid Transform  RotationMethod=RotationSequence  FollAlignAxisA=+X  BaseAlignAxisA=+Y  FollAlignAxisB=+Y  BaseAlignAxisB=+Z  RotationStandardAxis=+Z  RotationAngle=90  RotationAngleUnits=deg  RotationArbitraryAxis=[0 0 1]  RotationSequenceAxes=BaseAxes  RotationSequence=XYZ  RotationSequenceAngles=[-90 -90 0]  RotationSequenceAnglesUnits=deg  RotationMatrix=[1 0 0;0 1 0;0 0 1]  Quaternion=[1 0 0 0]  TranslationMethod=None  TranslationCartesianOffset=[0 0 0]  TranslationCartesianOffsetUnits=m  TranslationStandardAxis=+Z  TranslationStandardOffset=0  TranslationStandardOffsetUnits=m  TranslationROffset=0  TranslationROffsetUnits=m  TranslationThetaOffset=0  TranslationThetaOffsetUnits=deg  TranslationZOffset=0  TranslationZOffsetUnits=m
  Rigid Transform3 : sm_lib/Frames and Transforms/Rigid Transform  RotationMethod=RotationSequence  FollAlignAxisA=+X  BaseAlignAxisA=+Y  FollAlignAxisB=+Y  BaseAlignAxisB=+Z  RotationStandardAxis=+Z  RotationAngle=-90  RotationAngleUnits=deg  RotationArbitraryAxis=[0 0 1]  RotationSequenceAxes=BaseAxes  RotationSequence=YXZ  RotationSequenceAngles=[90 90 0]  RotationSequenceAnglesUnits=deg  RotationMatrix=[1 0 0;0 1 0;0 0 1]  Quaternion=[1 0 0 0]  TranslationMethod=None  TranslationCartesianOffset=[0 0 0]  TranslationCartesianOffsetUnits=m  TranslationStandardAxis=+Z  TranslationStandardOffset=0  TranslationStandardOffsetUnits=m  TranslationROffset=0  TranslationROffsetUnits=m  TranslationThetaOffset=0  TranslationThetaOffsetUnits=deg  TranslationZOffset=0  TranslationZOffsetUnits=m
  Rigid Transform4 : sm_lib/Frames and Transforms/Rigid Transform  RotationMethod=RotationSequence  FollAlignAxisA=+X  BaseAlignAxisA=+Y  FollAlignAxisB=+Y  BaseAlignAxisB=+Z  RotationStandardAxis=+Z  RotationAngle=90  RotationAngleUnits=deg  RotationArbitraryAxis=[0 0 1]  RotationSequenceAxes=BaseAxes  RotationSequence=XYZ  RotationSequenceAngles=[-90 -90 0]  RotationSequenceAnglesUnits=deg  RotationMatrix=[1 0 0;0 1 0;0 0 1]  Quaternion=[1 0 0 0]  TranslationMethod=None  TranslationCartesianOffset=[0 0 0]  TranslationCartesianOffsetUnits=m  TranslationStandardAxis=+Z  TranslationStandardOffset=0  TranslationStandardOffsetUnits=m  TranslationROffset=0  TranslationROffsetUnits=m  TranslationThetaOffset=0  TranslationThetaOffsetUnits=deg  TranslationZOffset=0  TranslationZOffsetUnits=m
  F : PMIOPort  Side=Left
  JF : PMIOPort  Port=2  Side=Left
  B : PMIOPort  Port=3  Side=Right
  JB : PMIOPort  Port=4  Side=Right
  connections:
  Rigid Transform1/LConn1 -- B/RConn1
  Rigid Transform2/RConn1 -- JB/RConn1
  Rigid Transform3/LConn1 -- JF/RConn1
  Rigid Transform4/RConn1 -- F/RConn1
  Rigid Transform1/RConn1 -- Linear Guide/RConn1
  Rigid Transform2/LConn1 -- Linear Guide/LConn1
  Rigid Transform3/RConn1 -- Carriage/RConn1
  Rigid Transform4/LConn1 -- Carriage/LConn1

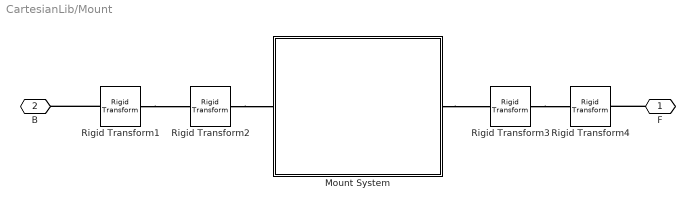
== system CartesianLib/Mount ==
  Mount System : Subsystem  Variant=on  VariantControlMode=label  LabelModeActiveChoice=PlateMount  mask{typeMount=Plate mount, widthMount=0.05, tMount=widthMount/8, angleMount=45, angleRotate=0}
      mask prompts: typeMount "Mount type"; widthMount "Mount width (m)"; tMount "Mount thickness (m)"; angleMount "Mount angle (deg)"; angleRotate "Rotation angle about mount base (deg)"
      mask Callback typeMount:
      | maskObj = Simulink.Mask.get(gcb);
      | typeMount = maskObj.getParameter('typeMount');
      | widthMount = maskObj.getParameter('widthMount');
      | tMount = maskObj.getParameter('tMount');
      | angleMount = maskObj.getParameter('angleMount');
      | angleRotate = maskObj.getParameter('angleRotate');
      | %mountSystemPath = [gcb,'/Mount System'];
      | if strcmp(typeMount.Value,'Plate mount')
      |     widthMount.Visible = 'on';
      |     tMount.Visible = 'on';
      |     angleMount.Visible = 'off';
      |     angleRotate.Visible = 'off';
      |     %set_param(mountSystemPath, 'LabelModeActiveChoice', 'PlateMount');
      | elseif strcmp(typeMount.Value,'L-shaped mount')
      |     widthMount.Visible = 'on';
      |     tMount.Visible = 'on';
      |     angleMount.Visible = 'off';
      |     angleRotate.Visible = 'on';
      |     %set_param(mountSystemPath, 'LabelModeActiveChoice', 'LMount');
      | elseif strcmp(typeMount.Value,'Angle mount')
      |     widthMount.Visible = 'on';
      |     tMount.Visible = 'on';
      |     angleMount.Visible = 'on';
      |     angleRotate.Visible = 'on';
      |     %set_param(mountSystemPath, 'LabelModeActiveChoice', 'AngleMount');
      | end
      mask TypeOptions angleMount: Angle Mount/angleMount
      mask TypeOptions angleRotate: L-Shaped Mount/angleRotate
  Rigid Transform2 : sm_lib/Frames and Transforms/Rigid Transform  RotationMethod=StandardAxis  FollAlignAxisA=+X  BaseAlignAxisA=+Y  FollAlignAxisB=+Y  BaseAlignAxisB=+Z  RotationStandardAxis=+Y  RotationAngle=angleRotate  RotationAngleUnits=deg  RotationArbitraryAxis=[0 0 1]  RotationSequenceAxes=BaseAxes  RotationSequence=XYZ  RotationSequenceAngles=[0 180 0]  RotationSequenceAnglesUnits=deg  RotationMatrix=[1 0 0;0 1 0;0 0 1]  Quaternion=[1 0 0 0]  TranslationMethod=None  TranslationCartesianOffset=[0 0 0]  TranslationCartesianOffsetUnits=m  TranslationStandardAxis=+Z  TranslationStandardOffset=0  TranslationStandardOffsetUnits=m  TranslationROffset=0  TranslationROffsetUnits=m  TranslationThetaOffset=0  TranslationThetaOffsetUnits=deg  TranslationZOffset=0  TranslationZOffsetUnits=m
  Rigid Transform3 : sm_lib/Frames and Transforms/Rigid Transform  RotationMethod=StandardAxis  FollAlignAxisA=+X  BaseAlignAxisA=+Y  FollAlignAxisB=+Y  BaseAlignAxisB=+Z  RotationStandardAxis=-Y  RotationAngle=angleRotate  RotationAngleUnits=deg  RotationArbitraryAxis=[0 0 1]  RotationSequenceAxes=BaseAxes  RotationSequence=ZYX  RotationSequenceAngles=[0 -180 0]  RotationSequenceAnglesUnits=deg  RotationMatrix=[1 0 0;0 1 0;0 0 1]  Quaternion=[1 0 0 0]  TranslationMethod=None  TranslationCartesianOffset=[0 0 0]  TranslationCartesianOffsetUnits=m  TranslationStandardAxis=+Z  TranslationStandardOffset=0  TranslationStandardOffsetUnits=m  TranslationROffset=0  TranslationROffsetUnits=m  TranslationThetaOffset=0  TranslationThetaOffsetUnits=deg  TranslationZOffset=0  TranslationZOffsetUnits=m
  Rigid Transform1 : sm_lib/Frames and Transforms/Rigid Transform  RotationMethod=RotationSequence  FollAlignAxisA=+X  BaseAlignAxisA=+Y  FollAlignAxisB=+Y  BaseAlignAxisB=+Z  RotationStandardAxis=+Y  RotationAngle=angleRotate  RotationAngleUnits=deg  RotationArbitraryAxis=[0 0 1]  RotationSequenceAxes=BaseAxes  RotationSequence=XYZ  RotationSequenceAngles=[0 0 0]  RotationSequenceAnglesUnits=deg  RotationMatrix=[1 0 0;0 1 0;0 0 1]  Quaternion=[1 0 0 0]  TranslationMethod=None  TranslationCartesianOffset=[0 0 0]  TranslationCartesianOffsetUnits=m  TranslationStandardAxis=+Z  TranslationStandardOffset=0  TranslationStandardOffsetUnits=m  TranslationROffset=0  TranslationROffsetUnits=m  TranslationThetaOffset=0  TranslationThetaOffsetUnits=deg  TranslationZOffset=0  TranslationZOffsetUnits=m
  Rigid Transform4 : sm_lib/Frames and Transforms/Rigid Transform  RotationMethod=RotationSequence  FollAlignAxisA=+X  BaseAlignAxisA=+Y  FollAlignAxisB=+Y  BaseAlignAxisB=+Z  RotationStandardAxis=-Y  RotationAngle=angleRotate  RotationAngleUnits=deg  RotationArbitraryAxis=[0 0 1]  RotationSequenceAxes=BaseAxes  RotationSequence=XYZ  RotationSequenceAngles=[0 0 0]  RotationSequenceAnglesUnits=deg  RotationMatrix=[1 0 0;0 1 0;0 0 1]  Quaternion=[1 0 0 0]  TranslationMethod=None  TranslationCartesianOffset=[0 0 0]  TranslationCartesianOffsetUnits=m  TranslationStandardAxis=+Z  TranslationStandardOffset=0  TranslationStandardOffsetUnits=m  TranslationROffset=0  TranslationROffsetUnits=m  TranslationThetaOffset=0  TranslationThetaOffsetUnits=deg  TranslationZOffset=0  TranslationZOffsetUnits=m
  F : PMIOPort  Side=Left
  B : PMIOPort  Port=2  Side=Right
  connections:
  Rigid Transform2/RConn1 -- Mount System/LConn1
  Rigid Transform3/RConn1 -- Rigid Transform4/LConn1
  Rigid Transform1/LConn1 -- B/RConn1
  F/RConn1 -- Rigid Transform4/RConn1
  Rigid Transform1/RConn1 -- Rigid Transform2/LConn1
  Mount System/RConn1 -- Rigid Transform3/LConn1

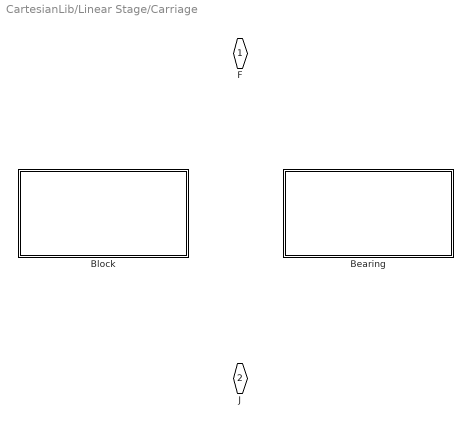
== system CartesianLib/Linear Stage/Carriage ==
  Bearing : Subsystem  VariantControl=Bearing  mask{lengthBearing=lengthBearing, widthBearing=widthBearing}
      mask prompts: lengthBearing "Bearing length (m)"; widthBearing "Bearing width (m)"
      mask init:
      | % Bearing box section
      | w = get_param(gcb,'value@widthBearing');
      | boxSection = [-w/2 w/2; -w/2 -w/2; w/2 -w/2; w/2 0];
      | 
      | % Adding annular area for shaft
      | theta = (pi/180)*[linspace(360,0,361)]';
      | r = 0.25*w; % Shaft radius (shaft diameter is designed to be half of bearing width)
      | circle = [r*cos(theta), r*sin(theta)];
      | bearingSection = [boxSection; circle];
      | bearingSection = [bearingSection; w/2 0; w/2 w/2];
      settings: PortSchema="{\"entries\":[{\"content\":{\"sides\":[{\"content\":{},\"type\":\"ConnectorPlacement.EquallySpacedRectSide\",\"uuid\":\"5b485af5-4f05-4248-a7f3-08377bf9cff2\"},{\"content\":{\"side\":\"RIGHT\"},\"type\":\"ConnectorPlacement.EquallySpacedRectSide\",\"uuid\":\"824380b3-967b-4422-aed9-09760effc9b4\"},{\"content\":{\"connectorIds\":[\"LConn1\"],\"side\":\"TOP\"},\"type\":\"ConnectorPlacement.EquallySpacedRectSide\",\"uuid\":\"4c7d634e-a270-49ee-a9b6-ce866eb97663\"},{\"content\":{\"connectorIds\":[\"RConn1\"],\"side\":\"BOTTOM\"},\"type\":\"ConnectorPlacement.EquallySpacedRectSide\",\"uuid\":\"4b6309f5-a0b1-41be-8c73-9bd13c5c2e87\"}]},\"type\":\"ConnectorPlacement.EquallySpacedConnector\",\"uuid\":\"704e5fa1-0bef-4b5b-a1a4-570354550c26\"}],\"packageUris\":[\"http://schema.mathworks.com/mf0/Connector/R2020b\"],\"version\":\"1.0\"}"
      mask Display:
      | image('BearingIcon.png');
      | port_label('rconn',1,'J');
      | port_label('lconn',1,'F');
  Block : Subsystem  VariantControl=Block  mask{lengthBlock=lengthBlock, widthSlideSurface=widthRail}
      mask prompts: lengthBlock "Block length (m)"; widthSlideSurface "Sliding surface width (m)"
      mask init:
      | % Vertices coordinates
      | v1 = [0.95*widthSlideSurface, 1.5*widthSlideSurface];
      | v2 = [-0.95*widthSlideSurface, 1.5*widthSlideSurface];
      | v3 = [-widthSlideSurface, 1.45*widthSlideSurface];
      | v4 = [-widthSlideSurface, 0.32*widthSlideSurface];
      | v5 = [-0.95*widthSlideSurface, 0.27*widthSlideSurface];
      | v6 = [-0.5*widthSlideSurface, 0.27*widthSlideSurface];
      | v7 = [-0.4*widthSlideSurface, 0.45*widthSlideSurface];
      | v8 = [-0.4*widthSlideSurface, 0.6*widthSlideSurface];
      | v9 = [-0.5*widthSlideSurface, 0.75*widthSlideSurface];
      | v10 = [-0.5*widthSlideSurface, 0.85*widthSlideSurface];
      | v11 = [-0.4*widthSlideSurface, widthSlideSurface];
      | v12 = [0.4*widthSlideSurface, widthSlideSurface];
      | v13 = [0.5*widthSlideSurface, 0.85*widthSlideSurface];
      | v14 = [0.5*widthSlideSurface, 0.75*widthSlideSurface];
      | v15 = [0.4*widthSlideSurface, 0.6*widthSlideSurface];
      | v16 = [0.4*widthSlideSurface, 0.45*widthSlideSurface];
      | v17 = [0.5*widthSlideSurface, 0.27*widthSlideSurface];
      | v18 = [0.95*widthSlideSurface, 0.27*widthSlideSurface];
      | v19 = [widthSlideSurface, 0.32*widthSlideSurface];
      | v20 = [widthSlideSurface, 1.45*widthSlideSurface];
      | sectionBlock = [v1; v2; v3; v4; v5; v6; v7; v8; v9; v10; v11; v12;...
      |     v13; v14; v15; v16; v17; v18; v19; v20];
      settings: PortSchema="{\"entries\":[{\"content\":{\"sides\":[{\"content\":{},\"type\":\"ConnectorPlacement.EquallySpacedRectSide\",\"uuid\":\"5b485af5-4f05-4248-a7f3-08377bf9cff2\"},{\"content\":{\"side\":\"RIGHT\"},\"type\":\"ConnectorPlacement.EquallySpacedRectSide\",\"uuid\":\"824380b3-967b-4422-aed9-09760effc9b4\"},{\"content\":{\"connectorIds\":[\"LConn1\"],\"side\":\"TOP\"},\"type\":\"ConnectorPlacement.EquallySpacedRectSide\",\"uuid\":\"4c7d634e-a270-49ee-a9b6-ce866eb97663\"},{\"content\":{\"connectorIds\":[\"RConn1\"],\"side\":\"BOTTOM\"},\"type\":\"ConnectorPlacement.EquallySpacedRectSide\",\"uuid\":\"b6590794-ed4a-45c8-9795-b62ea8052d06\"}]},\"type\":\"ConnectorPlacement.EquallySpacedConnector\",\"uuid\":\"704e5fa1-0bef-4b5b-a1a4-570354550c26\"}],\"packageUris\":[\"http://schema.mathworks.com/mf0/Connector/R2020b\"],\"version\":\"1.0\"}"
      mask Display:
      | image('BlockIcon.png');
      | port_label('rconn',1,'J');
      | port_label('lconn',1,'F');
  F : PMIOPort  Side=Left
  J : PMIOPort  Port=2  Side=Right

== system CartesianLib/Linear Stage/Linear Guide ==
  Lead Screw : Subsystem  VariantControl=Screw  mask{lengthScrew=lengthScrew, diaScrew=diaScrew}
      mask prompts: lengthScrew "Screw length (m)"; diaScrew "Screw diameter (m)"
      settings: PortSchema="{\"entries\":[{\"content\":{\"sides\":[{\"content\":{},\"type\":\"ConnectorPlacement.EquallySpacedRectSide\",\"uuid\":\"5b485af5-4f05-4248-a7f3-08377bf9cff2\"},{\"content\":{\"side\":\"RIGHT\"},\"type\":\"ConnectorPlacement.EquallySpacedRectSide\",\"uuid\":\"824380b3-967b-4422-aed9-09760effc9b4\"},{\"content\":{\"connectorIds\":[\"LConn1\"],\"side\":\"TOP\"},\"type\":\"ConnectorPlacement.EquallySpacedRectSide\",\"uuid\":\"4c7d634e-a270-49ee-a9b6-ce866eb97663\"},{\"content\":{\"connectorIds\":[\"RConn1\"],\"side\":\"BOTTOM\"},\"type\":\"ConnectorPlacement.EquallySpacedRectSide\",\"uuid\":\"3d224218-206f-49bf-9203-207f4ae7c9b3\"}]},\"type\":\"ConnectorPlacement.EquallySpacedConnector\",\"uuid\":\"704e5fa1-0bef-4b5b-a1a4-570354550c26\"}],\"packageUris\":[\"http://schema.mathworks.com/mf0/Connector/R2020b\"],\"version\":\"1.0\"}"
      mask Display:
      | image('LeadscrewIcon.png');
      | port_label('rconn',1,'B');
      | port_label('lconn',1,'J');
  Rail : Subsystem  VariantControl=Rail  mask{lengthRail=lengthRail, widthRail=widthRail}
      mask prompts: lengthRail "Rail length (m)"; widthRail "Rail width (m)"
      mask init:
      | % Vertices coordinates
      | v1 = [0.4*widthRail, widthRail];
      | v2 = [-0.4*widthRail, widthRail];
      | v3 = [-0.5*widthRail, 0.85*widthRail];
      | v4 = [-0.5*widthRail, 0.75*widthRail];
      | v5 = [-0.4*widthRail, 0.6*widthRail];
      | v6 = [-0.4*widthRail, 0.45*widthRail];
      | v7 = [-0.5*widthRail, 0.27*widthRail];
      | v8 = [-0.5*widthRail, 0.05*widthRail];
      | v9 = [-0.45*widthRail, 0];
      | v10 = [0.45*widthRail, 0];
      | v11 = [0.5*widthRail, 0.05*widthRail];
      | v12 = [0.5*widthRail, 0.27*widthRail];
      | v13 = [0.4*widthRail, 0.45*widthRail];
      | v14 = [0.4*widthRail, 0.6*widthRail];
      | v15 = [0.5*widthRail, 0.75*widthRail];
      | v16 = [0.5*widthRail, 0.85*widthRail];
      | sectionRail = [v1; v2; v3; v4; v5; v6; v7; v8; v9; v10; v11; v12; v13; v14; v15; v16];
      settings: PortSchema="{\"entries\":[{\"content\":{\"sides\":[{\"content\":{},\"type\":\"ConnectorPlacement.EquallySpacedRectSide\",\"uuid\":\"5b485af5-4f05-4248-a7f3-08377bf9cff2\"},{\"content\":{\"side\":\"RIGHT\"},\"type\":\"ConnectorPlacement.EquallySpacedRectSide\",\"uuid\":\"824380b3-967b-4422-aed9-09760effc9b4\"},{\"content\":{\"connectorIds\":[\"LConn1\"],\"side\":\"TOP\"},\"type\":\"ConnectorPlacement.EquallySpacedRectSide\",\"uuid\":\"4c7d634e-a270-49ee-a9b6-ce866eb97663\"},{\"content\":{\"connectorIds\":[\"RConn1\"],\"side\":\"BOTTOM\"},\"type\":\"ConnectorPlacement.EquallySpacedRectSide\",\"uuid\":\"bdc8e5c8-d37f-4730-b9ec-99442fb78d27\"}]},\"type\":\"ConnectorPlacement.EquallySpacedConnector\",\"uuid\":\"704e5fa1-0bef-4b5b-a1a4-570354550c26\"}],\"packageUris\":[\"http://schema.mathworks.com/mf0/Connector/R2020b\"],\"version\":\"1.0\"}"
      mask Display:
      | image('RailIcon.png')
      | port_label('rconn',1,'B');
      | port_label('lconn',1,'J');
  J : PMIOPort  Side=Left
  B : PMIOPort  Port=2  Side=Right
